simulink model "simulink_acados_vehicle_model"  (R2023b)
settings: Solver=FixedStepAuto  StartTime=0.0  StopTime=20  RelTol=1e-3
undefined symbols (not defined in the file or in its folder): d_delta_thd, lbx, N, Ts, ubx, V0, V_ref
settings Model: Creator=maart  LastModifiedBy=maart

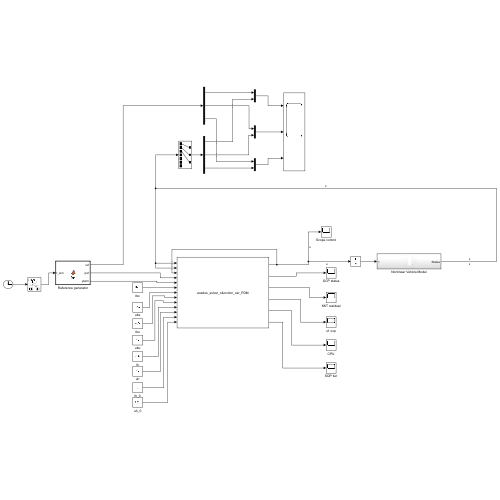
[thumbnail: Simulink's stored preview of the top-level diagram]
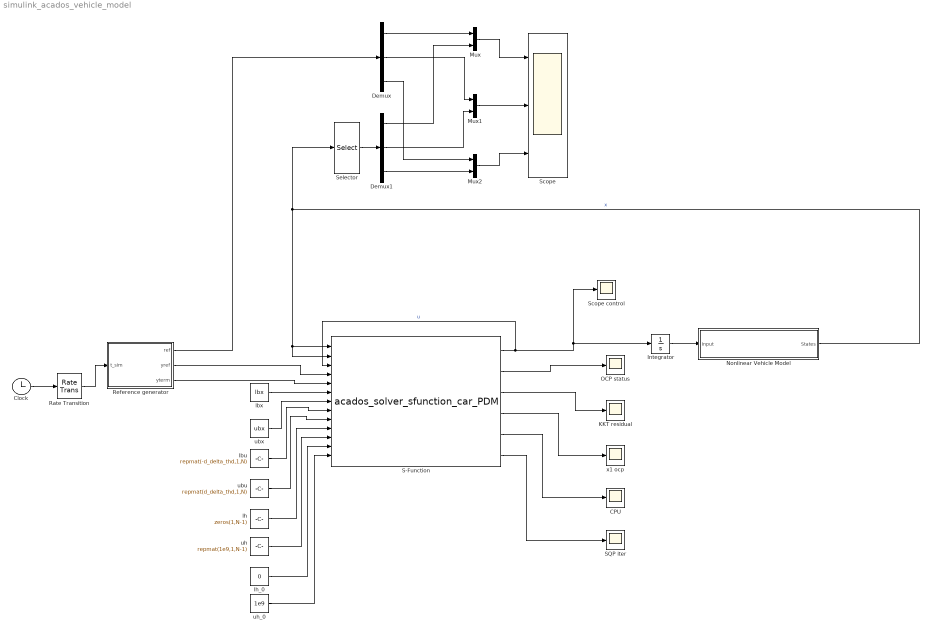
== system simulink_acados_vehicle_model ==
  CPU : Scope
      settings: Description=status
  Clock : Clock
  Demux : Demux  Outputs=3
  Demux1 : Demux  Outputs=3
  Integrator : Integrator
  KKT residual : Scope
      settings: Description=status
  Mux : Mux  Inputs=2
  Mux1 : Mux  Inputs=2
  Mux2 : Mux  Inputs=2
  Nonlinear Vehicle Model : Subsystem
  OCP status : Scope
      settings: Description=status
  Rate Transition : RateTransition
  Reference generator : MATLAB Function  TreatAsAtomicUnit=on
  S-Function : S-Function  FunctionName=acados_solver_sfunction_car_PDM  SFunctionDeploymentMode=off  EnableBusSupport=off
  SQP iter : Scope
      settings: Description=status
  Scope : Scope  NumInputPorts=3
  Scope control : Scope
  Selector : Selector  InputPortWidth=7  IndexOptions=Index vector (dialog)  Indices=[1:3]  OutputSizes=1
  lbu : Constant  Value=repmat(-d_delta_thd,1,N)
  lbx : Constant  Value=lbx
  lh : Constant  Value=zeros(1,N-1)
  lh_0 : Constant  Value=0
  ubu : Constant  Value=repmat(d_delta_thd,1,N)
  ubx : Constant  Value=ubx
  uh : Constant  Value=repmat(1e9,1,N-1)
  uh_0 : Constant  Value=1e9
  x1 ocp : Scope
      settings: Description=status
  wires:
  Rate Transition/1 -> Reference generator/1(t_sim)
  Nonlinear Vehicle Model/1(States) -> Selector/1, S-Function/2, S-Function/1  "x"
  Reference generator/3(yterm) -> S-Function/5
  S-Function/4 -> x1 ocp/1
  Clock/1 -> Rate Transition/1
  S-Function/1 -> Scope control/1, Integrator/1, S-Function/3  "u"
  Reference generator/2(yref) -> S-Function/4
  S-Function/3 -> KKT residual/1
  S-Function/6 -> SQP iter/1
  S-Function/2 -> OCP status/1
  S-Function/5 -> CPU/1
  Integrator/1 -> Nonlinear Vehicle Model/1(Input)
  Reference generator/1(ref) -> Demux/1
  Selector/1 -> Demux1/1
  Demux1/1 -> Mux/2
  Demux/1 -> Mux/1
  Demux1/2 -> Mux1/2
  Demux/2 -> Mux1/1
  Demux/3 -> Mux2/1
  Demux1/3 -> Mux2/2
  Mux2/1 -> Scope/3
  Mux1/1 -> Scope/2
  Mux/1 -> Scope/1
  lbx/1 -> S-Function/6
  ubx/1 -> S-Function/7
  lbu/1 -> S-Function/8
  ubu/1 -> S-Function/9
  lh/1 -> S-Function/10
  uh/1 -> S-Function/11
  lh_0/1 -> S-Function/12
  uh_0/1 -> S-Function/13

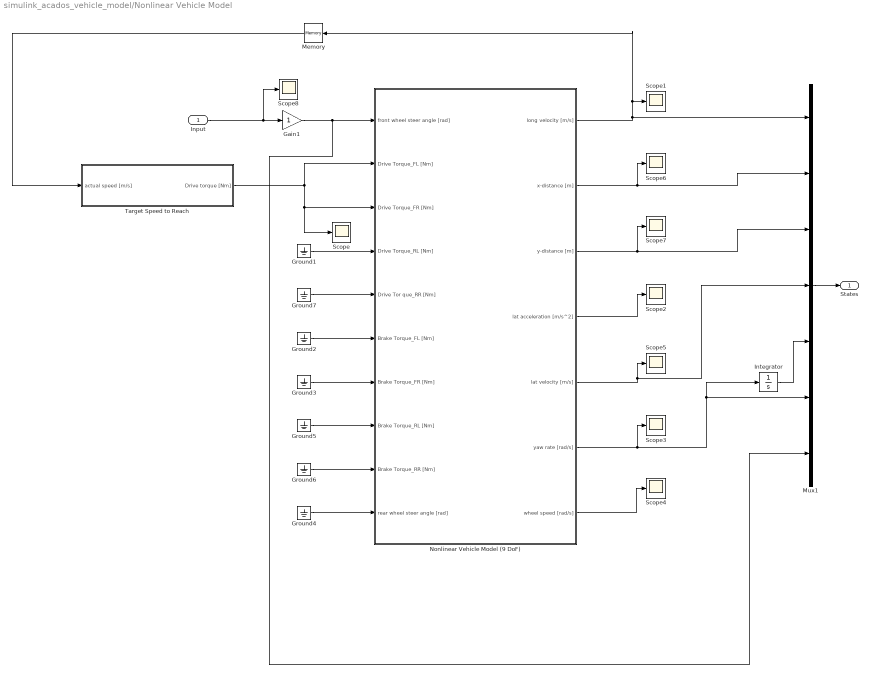
== system simulink_acados_vehicle_model/Nonlinear Vehicle Model ==
  Input : Inport
  Gain1 : Gain
  Ground{1..7} (7 alike) : Ground
  Integrator : Integrator
  Memory : Memory
  Mux1 : Mux  Inputs=7
  Nonlinear Vehicle Model (9 DoF) : Subsystem
      mask help: Simulink:masks:GenSFuncDesc_MD
      mask Help: eval('feval(''rtwprivate'',''rtwhelpview'',''rtw_sfcn_block'')');
  Scope{,1..8} (9 alike) : Scope
  Target Speed to Reach : Subsystem
  States : Outport
  wires:
  Nonlinear Vehicle Model (9 DoF)/2(x-distance [m]) -> Mux1/2, Scope6/1
  Input/1 -> Scope8/1, Gain1/1
  Nonlinear Vehicle Model (9 DoF)/5(lat velocity [m/s]) -> Scope5/1, Mux1/4
  Ground3/1 -> Nonlinear Vehicle Model (9 DoF)/7(Brake Torque_FR [Nm])
  Nonlinear Vehicle Model (9 DoF)/3(y-distance [m]) -> Mux1/3, Scope7/1
  Nonlinear Vehicle Model (9 DoF)/1(long velocity [m/s]) -> Memory/1, Scope1/1, Mux1/1
  Nonlinear Vehicle Model (9 DoF)/4(lat acceleration [m/s^2]) -> Scope2/1
  Nonlinear Vehicle Model (9 DoF)/6(yaw rate [rad/s]) -> Scope3/1, Mux1/6, Integrator/1
  Ground2/1 -> Nonlinear Vehicle Model (9 DoF)/6(Brake Torque_FL [Nm])
  Mux1/1 -> States/1
  Integrator/1 -> Mux1/5
  Ground4/1 -> Nonlinear Vehicle Model (9 DoF)/10(rear wheel steer angle [rad])
  Ground5/1 -> Nonlinear Vehicle Model (9 DoF)/8(Brake Torque_RL [Nm])
  Ground6/1 -> Nonlinear Vehicle Model (9 DoF)/9(Brake Torque_RR [Nm])
  Nonlinear Vehicle Model (9 DoF)/7(wheel speed [rad/s]) -> Scope4/1
  Target Speed to Reach/1(Drive torque [Nm]) -> Scope/1, Nonlinear Vehicle Model (9 DoF)/3(Drive Torque_FR [Nm]), Nonlinear Vehicle Model (9 DoF)/2(Drive Torque_FL [Nm])
  Gain1/1 -> Nonlinear Vehicle Model (9 DoF)/1(front wheel steer angle [rad]), Mux1/7
  Ground7/1 -> Nonlinear Vehicle Model (9 DoF)/5(Drive Tor	que_RR [Nm])
  Ground1/1 -> Nonlinear Vehicle Model (9 DoF)/4(Drive Torque_RL [Nm])
  Memory/1 -> Target Speed to Reach/1(actual speed [m/s])

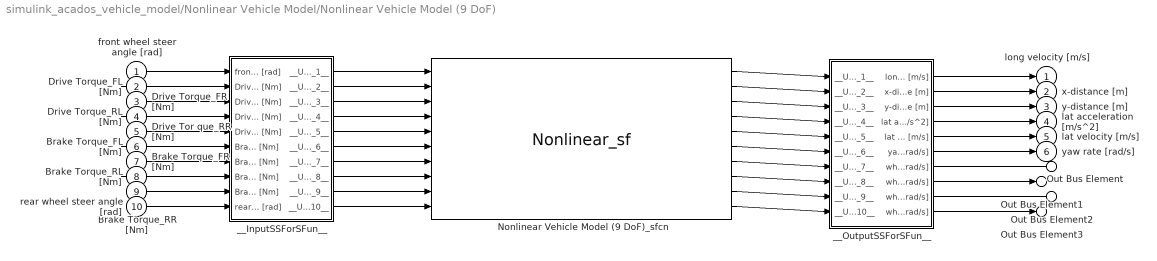
== system simulink_acados_vehicle_model/Nonlinear Vehicle Model/Nonlinear Vehicle Model (9 DoF) ==
  front wheel steer angle [rad] : Inport
  Drive Torque_FL [Nm] : Inport  Port=2
  Drive Torque_FR [Nm] : Inport  Port=3
  Drive Torque_RL [Nm] : Inport  Port=4
  Drive Tor	que_RR [Nm] : Inport  Port=5
  Brake Torque_FL [Nm] : Inport  Port=6
  Brake Torque_FR [Nm] : Inport  Port=7
  Brake Torque_RL [Nm] : Inport  Port=8
  Brake Torque_RR [Nm] : Inport  Port=9
  rear wheel steer angle [rad] : Inport  Port=10
  Nonlinear Vehicle Model (9 DoF)_sfcn : S-Function  FunctionName=Nonlinear_sf  SFunctionModules=""  SFunctionDeploymentMode=off  EnableBusSupport=off  mask{rtw_sf_name=Nonlinear_sf, showVar=off}
      mask prompts: rtw_sf_name "Simulink:masks:GenSFuncName_MP"; showVar "Simulink:masks:GenSFuncShowModuleList_MP"
      mask help: Simulink:masks:GenSFuncDesc_MD
      mask init:
      | displist = '';
      | if ~strcmp(get_param(gcb, 'FunctionName'), rtw_sf_name);
      |   set_param(gcb, 'FunctionName', rtw_sf_name);
      | end
      | % Check if we are generating code
      | rtw_mode = false;
      | if strcmpi(get_param(bdroot(gcb),'SimulationStatus'),'Initializing')
      | 	rtw_mode = strcmpi(get_param(bdroot(gcb),'BuildingRTWCode'),'on') && ...
      | 		~strcmpi(get_param(bdroot(gcb),'TargetStyle'),'SimulationTarget');
      | end
      | if showVar || rtw_mode
      | 	if exist('rtwsfunc') == 2 | exist('rtwsfunc') == 6
      | 		tmplist = rtwsfunc(rtw_sf_name,gcb);
      | 		tmplist = DAStudio.message('Simulink:masks:GenSFuncListOfModules_IC', tmplist);
      | 	elseif showVar
      | 		tmplist1 = DAStudio.message('Simulink:masks:GenSFuncListOfModules_IC', '');
      |         tmplist2 = DAStudio.message('Simulink:masks:GenSFuncNotLicensed_IC');
      |         tmplist = [tmplist1 tmplist2];
      |  	end
      | end
      | if showVar
      |   displist = tmplist;
      | end
      settings: CopyFcn=|
      | if ~strcmp(get_param(gcb,'Linkstatus'),'none') && ...
      | ~strcmp(get_param(gcb,'Linkstatus'),'implicit')
      |   set_param(gcb,'LinkStatus','none');
      | end
      mask Help: eval('feval(''rtwprivate'',''rtwhelpview'',''rtw_sfcn_block'')');
      mask Display:
      | port_label('input',1,'front wheel steer angle [rad]');
      | port_label('input',2,'Drive Torque_FL [Nm]');
      | port_label('input',3,'Drive Torque_FR [Nm]');
      | port_label('input',4,'Drive Torque_RL [Nm]');
      | port_label('input',5,'Drive Tor	que_RR [Nm]');
      | port_label('input',6,'Brake Torque_FL [Nm]');
      | port_label('input',7,'Brake Torque_FR [Nm]');
      | port_label('input',8,'Brake Torque_RL [Nm]');
      | port_label('input',9,'Brake Torque_RR [Nm]');
      | port_label('input',10,'rear wheel steer angle [rad]');
      | port_label('output',1,'long velocity [m/s]');
      | port_label('output',2,'x-distance [m]');
      | port_label('output',3,'y-distance [m]');
      | port_label('output',4,'lat acceleration [m/s^2]');
      | port_label('output',5,'lat velocity [m/s]');
      | port_label('output',6,'yaw rate [rad/s]');
      | port_label('output',7,'wheel speed FL [rad/s]');
      | port_label('output',8,'wheel speed FR [rad/s]');
      | port_label('output',9,'wheel speed RL [rad/s]');
      | port_label('output',10,'wheel speed RR [rad/s]');
  __InputSSForSFun__ : Subsystem
  __OutputSSForSFun__ : Subsystem
  long velocity [m/s] : Outport  VectorParamsAs1DForOutWhenUnconnected=off
  x-distance [m] : Outport  Port=2  VectorParamsAs1DForOutWhenUnconnected=off
  y-distance [m] : Outport  Port=3  VectorParamsAs1DForOutWhenUnconnected=off
  lat acceleration [m/s^2] : Outport  Port=4  VectorParamsAs1DForOutWhenUnconnected=off
  lat velocity [m/s] : Outport  Port=5  VectorParamsAs1DForOutWhenUnconnected=off
  yaw rate [rad/s] : Outport  Port=6  VectorParamsAs1DForOutWhenUnconnected=off
  Out Bus Element : Outport  Port=7  PortName=wheel speed [rad/s]  Element=wheel speed FL [rad/s]
  Out Bus Element1 : Outport  Port=7  PortName=wheel speed [rad/s]  Element=wheel speed FR [rad/s]
  Out Bus Element2 : Outport  Port=7  PortName=wheel speed [rad/s]  Element=wheel speed RL [rad/s]
  Out Bus Element3 : Outport  Port=7  PortName=wheel speed [rad/s]  Element=wheel speed RR [rad/s]
  wires:
  front wheel steer angle [rad]/1 -> __InputSSForSFun__/1(front wheel steer angle [rad])
  Drive Torque_FL [Nm]/1 -> __InputSSForSFun__/2(Drive Torque_FL [Nm])
  Drive Torque_FR [Nm]/1 -> __InputSSForSFun__/3(Drive Torque_FR [Nm])
  Drive Torque_RL [Nm]/1 -> __InputSSForSFun__/4(Drive Torque_RL [Nm])
  Drive Tor	que_RR [Nm]/1 -> __InputSSForSFun__/5(Drive Tor	que_RR [Nm])
  Brake Torque_FL [Nm]/1 -> __InputSSForSFun__/6(Brake Torque_FL [Nm])
  Brake Torque_FR [Nm]/1 -> __InputSSForSFun__/7(Brake Torque_FR [Nm])
  Brake Torque_RL [Nm]/1 -> __InputSSForSFun__/8(Brake Torque_RL [Nm])
  Brake Torque_RR [Nm]/1 -> __InputSSForSFun__/9(Brake Torque_RR [Nm])
  rear wheel steer angle [rad]/1 -> __InputSSForSFun__/10(rear wheel steer angle [rad])
  __InputSSForSFun__/1(__UniqueOutportName__1__) -> Nonlinear Vehicle Model (9 DoF)_sfcn/1
  __InputSSForSFun__/2(__UniqueOutportName__2__) -> Nonlinear Vehicle Model (9 DoF)_sfcn/2
  __InputSSForSFun__/3(__UniqueOutportName__3__) -> Nonlinear Vehicle Model (9 DoF)_sfcn/3
  __InputSSForSFun__/4(__UniqueOutportName__4__) -> Nonlinear Vehicle Model (9 DoF)_sfcn/4
  __InputSSForSFun__/5(__UniqueOutportName__5__) -> Nonlinear Vehicle Model (9 DoF)_sfcn/5
  __InputSSForSFun__/6(__UniqueOutportName__6__) -> Nonlinear Vehicle Model (9 DoF)_sfcn/6
  __InputSSForSFun__/7(__UniqueOutportName__7__) -> Nonlinear Vehicle Model (9 DoF)_sfcn/7
  __InputSSForSFun__/8(__UniqueOutportName__8__) -> Nonlinear Vehicle Model (9 DoF)_sfcn/8
  __InputSSForSFun__/9(__UniqueOutportName__9__) -> Nonlinear Vehicle Model (9 DoF)_sfcn/9
  __InputSSForSFun__/10(__UniqueOutportName__10__) -> Nonlinear Vehicle Model (9 DoF)_sfcn/10
  Nonlinear Vehicle Model (9 DoF)_sfcn/1 -> __OutputSSForSFun__/1(__UniqueInportName__1__)
  Nonlinear Vehicle Model (9 DoF)_sfcn/2 -> __OutputSSForSFun__/2(__UniqueInportName__2__)
  Nonlinear Vehicle Model (9 DoF)_sfcn/3 -> __OutputSSForSFun__/3(__UniqueInportName__3__)
  Nonlinear Vehicle Model (9 DoF)_sfcn/4 -> __OutputSSForSFun__/4(__UniqueInportName__4__)
  Nonlinear Vehicle Model (9 DoF)_sfcn/5 -> __OutputSSForSFun__/5(__UniqueInportName__5__)
  Nonlinear Vehicle Model (9 DoF)_sfcn/6 -> __OutputSSForSFun__/6(__UniqueInportName__6__)
  Nonlinear Vehicle Model (9 DoF)_sfcn/7 -> __OutputSSForSFun__/7(__UniqueInportName__7__)
  Nonlinear Vehicle Model (9 DoF)_sfcn/8 -> __OutputSSForSFun__/8(__UniqueInportName__8__)
  Nonlinear Vehicle Model (9 DoF)_sfcn/9 -> __OutputSSForSFun__/9(__UniqueInportName__9__)
  Nonlinear Vehicle Model (9 DoF)_sfcn/10 -> __OutputSSForSFun__/10(__UniqueInportName__10__)
  __OutputSSForSFun__/1(long velocity [m/s]) -> long velocity [m/s]/1
  __OutputSSForSFun__/2(x-distance [m]) -> x-distance [m]/1
  __OutputSSForSFun__/3(y-distance [m]) -> y-distance [m]/1
  __OutputSSForSFun__/4(lat acceleration [m/s^2]) -> lat acceleration [m/s^2]/1
  __OutputSSForSFun__/5(lat velocity [m/s]) -> lat velocity [m/s]/1
  __OutputSSForSFun__/6(yaw rate [rad/s]) -> yaw rate [rad/s]/1
  __OutputSSForSFun__/7(wheel speed FL [rad/s]) -> Out Bus Element/1
  __OutputSSForSFun__/8(wheel speed FR [rad/s]) -> Out Bus Element1/1
  __OutputSSForSFun__/9(wheel speed RL [rad/s]) -> Out Bus Element2/1
  __OutputSSForSFun__/10(wheel speed RR [rad/s]) -> Out Bus Element3/1

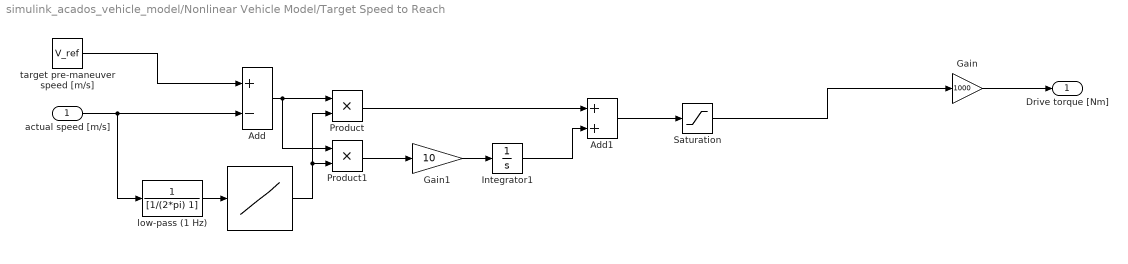
== system simulink_acados_vehicle_model/Nonlinear Vehicle Model/Target Speed to Reach ==
  actual speed [m/s] : Inport
  " " : Lookup_n-D  NumberOfTableDimensions=1  BreakpointsForDimension1="[-10  0  10 30]"  IndexSearchMethod=Linear search  Table=[0.1 0.1 1 1]  ExtrapMethod=Clip  RemoveProtectionInput=on  UseLastTableValue=on  RndMeth=Simplest
  Add : Sum  Inputs=+-
  Add1 : Sum
  Gain : Gain  Gain=1000
  Gain1 : Gain  Gain=10
  Integrator1 : Integrator  LimitOutput=on  UpperSaturationLimit=0.1  LowerSaturationLimit=-0.1
  Product : Product  RndMeth=Zero
  Product1 : Product  RndMeth=Zero
  Saturation : Saturate  UpperLimit=1  LowerLimit=0
  low-pass (1 Hz) : TransferFcn  Denominator=[1/(2*pi) 1]
  "target pre-maneuver speed [m/s] " : Constant  Value=V_ref
  Drive torque [Nm] : Outport
  wires:
  actual speed [m/s]/1 -> low-pass (1 Hz)/1, Add/2
  "target pre-maneuver speed [m/s] "/1 -> Add/1
  Gain1/1 -> Integrator1/1
  Product/1 -> Add1/1
  Add/1 -> Product/1, Product1/1
  Product1/1 -> Gain1/1
  " "/1 -> Product1/2, Product/2
  low-pass (1 Hz)/1 -> " "/1
  Add1/1 -> Saturation/1
  Integrator1/1 -> Add1/2
  Saturation/1 -> Gain/1
  Gain/1 -> Drive torque [Nm]/1

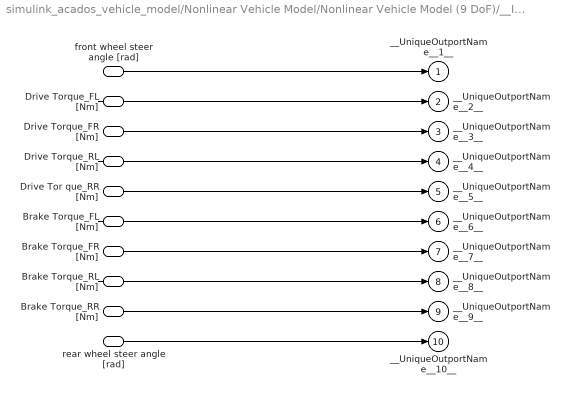
== system simulink_acados_vehicle_model/Nonlinear Vehicle Model/Nonlinear Vehicle Model (9 DoF)/__InputSSForSFun__ ==
  front wheel steer angle [rad] : Inport
  Drive Torque_FL [Nm] : Inport  Port=2
  Drive Torque_FR [Nm] : Inport  Port=3
  Drive Torque_RL [Nm] : Inport  Port=4
  Drive Tor	que_RR [Nm] : Inport  Port=5
  Brake Torque_FL [Nm] : Inport  Port=6
  Brake Torque_FR [Nm] : Inport  Port=7
  Brake Torque_RL [Nm] : Inport  Port=8
  Brake Torque_RR [Nm] : Inport  Port=9
  rear wheel steer angle [rad] : Inport  Port=10
  __UniqueOutportName__1__ : Outport
  __UniqueOutportName__2__ : Outport  Port=2
  __UniqueOutportName__3__ : Outport  Port=3
  __UniqueOutportName__4__ : Outport  Port=4
  __UniqueOutportName__5__ : Outport  Port=5
  __UniqueOutportName__6__ : Outport  Port=6
  __UniqueOutportName__7__ : Outport  Port=7
  __UniqueOutportName__8__ : Outport  Port=8
  __UniqueOutportName__9__ : Outport  Port=9
  __UniqueOutportName__10__ : Outport  Port=10
  wires:
  front wheel steer angle [rad]/1 -> __UniqueOutportName__1__/1
  Drive Torque_FL [Nm]/1 -> __UniqueOutportName__2__/1
  Drive Torque_FR [Nm]/1 -> __UniqueOutportName__3__/1
  Drive Torque_RL [Nm]/1 -> __UniqueOutportName__4__/1
  Drive Tor	que_RR [Nm]/1 -> __UniqueOutportName__5__/1
  Brake Torque_FL [Nm]/1 -> __UniqueOutportName__6__/1
  Brake Torque_FR [Nm]/1 -> __UniqueOutportName__7__/1
  Brake Torque_RL [Nm]/1 -> __UniqueOutportName__8__/1
  Brake Torque_RR [Nm]/1 -> __UniqueOutportName__9__/1
  rear wheel steer angle [rad]/1 -> __UniqueOutportName__10__/1

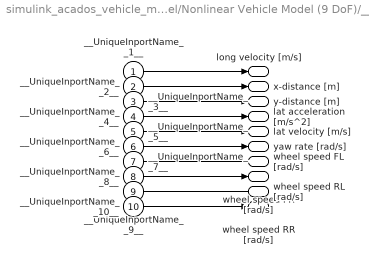
== system simulink_acados_vehicle_model/Nonlinear Vehicle Model/Nonlinear Vehicle Model (9 DoF)/__OutputSSForSFun__ ==
  __UniqueInportName__1__ : Inport
  __UniqueInportName__2__ : Inport  Port=2
  __UniqueInportName__3__ : Inport  Port=3
  __UniqueInportName__4__ : Inport  Port=4
  __UniqueInportName__5__ : Inport  Port=5
  __UniqueInportName__6__ : Inport  Port=6
  __UniqueInportName__7__ : Inport  Port=7
  __UniqueInportName__8__ : Inport  Port=8
  __UniqueInportName__9__ : Inport  Port=9
  __UniqueInportName__10__ : Inport  Port=10
  long velocity [m/s] : Outport  VectorParamsAs1DForOutWhenUnconnected=off
  x-distance [m] : Outport  Port=2  VectorParamsAs1DForOutWhenUnconnected=off
  y-distance [m] : Outport  Port=3  VectorParamsAs1DForOutWhenUnconnected=off
  lat acceleration [m/s^2] : Outport  Port=4  VectorParamsAs1DForOutWhenUnconnected=off
  lat velocity [m/s] : Outport  Port=5  VectorParamsAs1DForOutWhenUnconnected=off
  yaw rate [rad/s] : Outport  Port=6  VectorParamsAs1DForOutWhenUnconnected=off
  wheel speed FL [rad/s] : Outport  Port=7  VectorParamsAs1DForOutWhenUnconnected=off
  wheel speed FR [rad/s] : Outport  Port=8  VectorParamsAs1DForOutWhenUnconnected=off
  wheel speed RL [rad/s] : Outport  Port=9  VectorParamsAs1DForOutWhenUnconnected=off
  wheel speed RR [rad/s] : Outport  Port=10  VectorParamsAs1DForOutWhenUnconnected=off
  wires:
  __UniqueInportName__1__/1 -> long velocity [m/s]/1
  __UniqueInportName__2__/1 -> x-distance [m]/1
  __UniqueInportName__3__/1 -> y-distance [m]/1
  __UniqueInportName__4__/1 -> lat acceleration [m/s^2]/1
  __UniqueInportName__5__/1 -> lat velocity [m/s]/1
  __UniqueInportName__6__/1 -> yaw rate [rad/s]/1
  __UniqueInportName__7__/1 -> wheel speed FL [rad/s]/1
  __UniqueInportName__8__/1 -> wheel speed FR [rad/s]/1
  __UniqueInportName__9__/1 -> wheel speed RL [rad/s]/1
  __UniqueInportName__10__/1 -> wheel speed RR [rad/s]/1

== matlab function simulink_acados_vehicle_model/Reference generator ==
  data: ref output; yref output; t_sim input size=1; yterm output; V0 parameter size=1; N parameter size=1; Ts parameter size=1
function [ref,yref,yterm] = fcn(t_sim, V0, N, Ts)

    % t = t_sim + Ts*(1:N);
    % 
    % [~, Xp_ref, Yp_ref] = reference_corner(V0, t);
    % 
    % if length(Xp_ref) == 1
    %     Xp_ref = repmat(Xp_ref,1,N); 
    % end
    % 
    % if length(Yp_ref) == 1
    %     Yp_ref = repmat(Yp_ref,1,N);
    % end
    % 
    % arrayV0 = repmat(V0,1,N-1);
    % array0 = zeros(5,N-1);
    % 
    % yref = zeros(1,312);
    % yterm = zeros(1,7);
    % 
    % yref = reshape([arrayV0;Xp_ref(1:end-1);Yp_ref(1:end-1);array0],1,[]);
    % 
    % yterm = [V0;Xp_ref(end);Yp_ref(end);array0(:,1)];

    yref = zeros(1,8*(N-1));

    for i=1:N-1
        t = t_sim + Ts*(i-1);

        [~, Xp_ref, Yp_ref] = reference_corner(V0, t);

        yref(1+8*(i-1):8*(i-1)+8) = [V0;Xp_ref;Yp_ref;zeros(5,1)];

    end

    [~, Xp_ref, Yp_ref] = reference_corner(V0, (t_sim + Ts*N));

    yterm = [V0;Xp_ref;Yp_ref;zeros(4,1)];

    ref = yref(1:3);
